simulink model "SpheroMoveToPoint"  (R2014a)
settings: Solver=ode45  StartTime=0.0  StopTime=8  RelTol=1e-3
InitFcn:
  | sphName = uint8('Sphero-PGP');
StopFcn:
  | move(sphName, 0, 0)
  | move(sphName, 0, 0, 0)
undefined symbols (not defined in the file or in its folder): Kd, Ki, Kp
libraries: simulink x5, utility x1
settings Model: Creator=dsethi  LastModifiedBy=dsethi

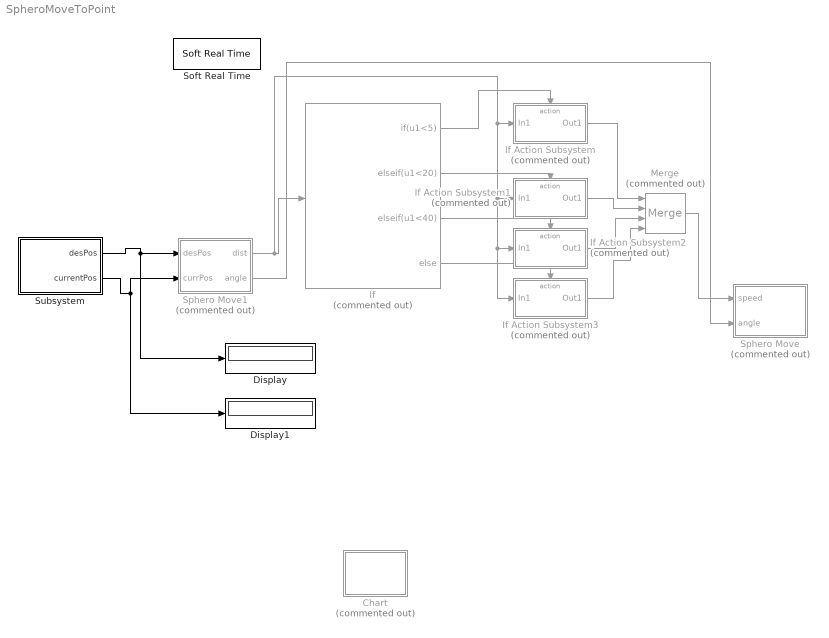
== system SpheroMoveToPoint ==
  Chart : Stateflow chart  Commented=on  TreatAsAtomicUnit=on
  Display : Display
  Display1 : Display
  If : If  Commented=on  IfExpression=u1<5  ElseIfExpressions=u1<20, u1<40
  If Action Subsystem : Subsystem  Commented=on  TreatAsAtomicUnit=on  mask{Kp=0, Ki=0, Kd=0}
  If Action Subsystem1 : Subsystem  Commented=on  TreatAsAtomicUnit=on  mask{Kp=4, Ki=0, Kd=0}
  If Action Subsystem2 : Subsystem  Commented=on  TreatAsAtomicUnit=on  mask{Kp=2, Ki=0, Kd=0}
  If Action Subsystem3 : Subsystem  Commented=on  TreatAsAtomicUnit=on  mask{Kp=0.5, Ki=0, Kd=0}
  Merge : Merge  Commented=on  Inputs=4
  Soft Real Time : utility/Soft Real Time  x=1
  Sphero Move : MATLAB Function  Commented=on  TreatAsAtomicUnit=on
  Sphero Move1 : MATLAB Function  Commented=on  TreatAsAtomicUnit=on
  Subsystem : Subsystem  mask{cameraNum=Logitech, desPos=[0, 0]}
      mask prompts: cameraNum "Camera"; desPos "Desired position (x, y coordinates)"
      mask init:
      | desPos = [0, 0]
      mask TypeOptions cameraNum: Logitech | Microsoft
  wires:
  Subsystem/1(desPos) -> Display/1, Sphero Move1/1(desPos)
  Subsystem/2(currentPos) -> Display1/1, Sphero Move1/2(currPos)
  Sphero Move1/2(angle) -> Sphero Move/2(angle)
  Sphero Move1/1(dist) -> If Action Subsystem1/1(In1), If Action Subsystem2/1(In1), If Action Subsystem3/1(In1), If Action Subsystem/1(In1), If/1
  If/1 -> If Action Subsystem/Action
  If/2 -> If Action Subsystem1/Action
  If/3 -> If Action Subsystem2/Action
  If/4 -> If Action Subsystem3/Action
  If Action Subsystem3/1(Out1) -> Merge/4
  If Action Subsystem2/1(Out1) -> Merge/3
  If Action Subsystem1/1(Out1) -> Merge/2
  If Action Subsystem/1(Out1) -> Merge/1
  Merge/1 -> Sphero Move/1(speed)

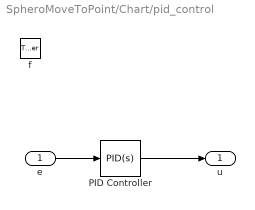
== system SpheroMoveToPoint/Chart/pid_control ==
  e : Inport  OutDataTypeStr=double  PortDimensions=1
  f : TriggerPort  TriggerType=function-call
      settings: CopyFcn=Stateflow.SLINSF.SimulinkMan.removeBlockPreDeleteFcn  PreDeleteFcn=Stateflow.SLINSF.SimulinkMan.unsafePredeleteFcn
  PID Controller : simulink/Continuous/PID Controller  Controller=PID  TimeDomain=Continuous-time  SampleTime=1  IntegratorMethod=Forward Euler  FilterMethod=Forward Euler  Form=Parallel  P=Kp  I=Ki  D=Kd  N=100  InitialConditionSource=internal  InitialConditionForIntegrator=0  InitialConditionForFilter=0  ExternalReset=none  LimitOutput=off  UpperSaturationLimit=inf  LowerSaturationLimit=-inf  LinearizeAsGain=on  AntiWindupMode=none  Kb=1  TrackingMode=off  Kt=1  PParamMin=[]  PParamMax=[]  IParamMin=[]  IParamMax=[]  DParamMin=[]  DParamMax=[]  NParamMin=[]  NParamMax=[]  KbParamMin=[]  KbParamMax=[]  KtParamMin=[]  KtParamMax=[]  POutMin=[]  POutMax=[]  IOutMin=[]  IOutMax=[]  DOutMin=[]  DOutMax=[]  NOutMin=[]  NOutMax=[]  KbOutMin=[]  KbOutMax=[]  KtOutMin=[]  KtOutMax=[]  IntegratorOutMin=[]  IntegratorOutMax=[]  FilterOutMin=[]  FilterOutMax=[]  SumOutMin=[]  SumOutMax=[]  SumI1OutMin=[]  SumI1OutMax=[]  SumI2OutMin=[]  SumI2OutMax=[]  SumI3OutMin=[]  SumI3OutMax=[]  SumDOutMin=[]  SumDOutMax=[]  SaturationOutMin=[]  SaturationOutMax=[]  IntegratorContinuousStateAttributes=''  IntegratorStateMustResolveToSignalObject=off  IntegratorRTWStateStorageClass=Auto  FilterContinuousStateAttributes=''  FilterStateMustResolveToSignalObject=off  FilterRTWStateStorageClass=Auto
  u : Outport
  wires:
  e/1 -> PID Controller/1
  PID Controller/1 -> u/1

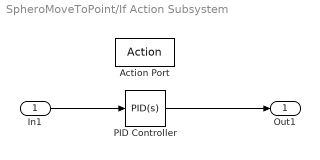
== system SpheroMoveToPoint/If Action Subsystem ==
  In1 : Inport
  Action Port : ActionPort  ActionType=then
  PID Controller : simulink/Continuous/PID Controller  Controller=PID  TimeDomain=Continuous-time  SampleTime=1  IntegratorMethod=Forward Euler  FilterMethod=Forward Euler  Form=Parallel  P=Kp  I=Ki  D=Kd  N=100  InitialConditionSource=internal  InitialConditionForIntegrator=0  InitialConditionForFilter=0  ExternalReset=none  LimitOutput=off  UpperSaturationLimit=inf  LowerSaturationLimit=-inf  LinearizeAsGain=on  AntiWindupMode=none  Kb=1  TrackingMode=off  Kt=1  PParamMin=[]  PParamMax=[]  IParamMin=[]  IParamMax=[]  DParamMin=[]  DParamMax=[]  NParamMin=[]  NParamMax=[]  KbParamMin=[]  KbParamMax=[]  KtParamMin=[]  KtParamMax=[]  POutMin=[]  POutMax=[]  IOutMin=[]  IOutMax=[]  DOutMin=[]  DOutMax=[]  NOutMin=[]  NOutMax=[]  KbOutMin=[]  KbOutMax=[]  KtOutMin=[]  KtOutMax=[]  IntegratorOutMin=[]  IntegratorOutMax=[]  FilterOutMin=[]  FilterOutMax=[]  SumOutMin=[]  SumOutMax=[]  SumI1OutMin=[]  SumI1OutMax=[]  SumI2OutMin=[]  SumI2OutMax=[]  SumI3OutMin=[]  SumI3OutMax=[]  SumDOutMin=[]  SumDOutMax=[]  SaturationOutMin=[]  SaturationOutMax=[]  IntegratorContinuousStateAttributes=''  IntegratorStateMustResolveToSignalObject=off  IntegratorRTWStateStorageClass=Auto  FilterContinuousStateAttributes=''  FilterStateMustResolveToSignalObject=off  FilterRTWStateStorageClass=Auto
  Out1 : Outport
  wires:
  PID Controller/1 -> Out1/1
  In1/1 -> PID Controller/1

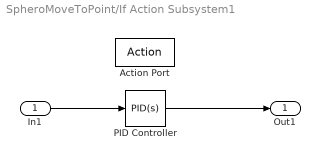
== system SpheroMoveToPoint/If Action Subsystem1 ==
  In1 : Inport
  Action Port : ActionPort  ActionType=elseif
  PID Controller : simulink/Continuous/PID Controller  Controller=PID  TimeDomain=Continuous-time  SampleTime=1  IntegratorMethod=Forward Euler  FilterMethod=Forward Euler  Form=Parallel  P=Kp  I=Ki  D=Kd  N=100  InitialConditionSource=internal  InitialConditionForIntegrator=0  InitialConditionForFilter=0  ExternalReset=none  LimitOutput=off  UpperSaturationLimit=inf  LowerSaturationLimit=-inf  LinearizeAsGain=on  AntiWindupMode=none  Kb=1  TrackingMode=off  Kt=1  PParamMin=[]  PParamMax=[]  IParamMin=[]  IParamMax=[]  DParamMin=[]  DParamMax=[]  NParamMin=[]  NParamMax=[]  KbParamMin=[]  KbParamMax=[]  KtParamMin=[]  KtParamMax=[]  POutMin=[]  POutMax=[]  IOutMin=[]  IOutMax=[]  DOutMin=[]  DOutMax=[]  NOutMin=[]  NOutMax=[]  KbOutMin=[]  KbOutMax=[]  KtOutMin=[]  KtOutMax=[]  IntegratorOutMin=[]  IntegratorOutMax=[]  FilterOutMin=[]  FilterOutMax=[]  SumOutMin=[]  SumOutMax=[]  SumI1OutMin=[]  SumI1OutMax=[]  SumI2OutMin=[]  SumI2OutMax=[]  SumI3OutMin=[]  SumI3OutMax=[]  SumDOutMin=[]  SumDOutMax=[]  SaturationOutMin=[]  SaturationOutMax=[]  IntegratorContinuousStateAttributes=''  IntegratorStateMustResolveToSignalObject=off  IntegratorRTWStateStorageClass=Auto  FilterContinuousStateAttributes=''  FilterStateMustResolveToSignalObject=off  FilterRTWStateStorageClass=Auto
  Out1 : Outport
  wires:
  In1/1 -> PID Controller/1
  PID Controller/1 -> Out1/1

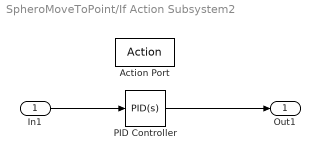
== system SpheroMoveToPoint/If Action Subsystem2 ==
  In1 : Inport
  Action Port : ActionPort  ActionType=elseif
  PID Controller : simulink/Continuous/PID Controller  Controller=PID  TimeDomain=Continuous-time  SampleTime=1  IntegratorMethod=Forward Euler  FilterMethod=Forward Euler  Form=Parallel  P=Kp  I=Ki  D=Kd  N=100  InitialConditionSource=internal  InitialConditionForIntegrator=0  InitialConditionForFilter=0  ExternalReset=none  LimitOutput=off  UpperSaturationLimit=inf  LowerSaturationLimit=-inf  LinearizeAsGain=on  AntiWindupMode=none  Kb=1  TrackingMode=off  Kt=1  PParamMin=[]  PParamMax=[]  IParamMin=[]  IParamMax=[]  DParamMin=[]  DParamMax=[]  NParamMin=[]  NParamMax=[]  KbParamMin=[]  KbParamMax=[]  KtParamMin=[]  KtParamMax=[]  POutMin=[]  POutMax=[]  IOutMin=[]  IOutMax=[]  DOutMin=[]  DOutMax=[]  NOutMin=[]  NOutMax=[]  KbOutMin=[]  KbOutMax=[]  KtOutMin=[]  KtOutMax=[]  IntegratorOutMin=[]  IntegratorOutMax=[]  FilterOutMin=[]  FilterOutMax=[]  SumOutMin=[]  SumOutMax=[]  SumI1OutMin=[]  SumI1OutMax=[]  SumI2OutMin=[]  SumI2OutMax=[]  SumI3OutMin=[]  SumI3OutMax=[]  SumDOutMin=[]  SumDOutMax=[]  SaturationOutMin=[]  SaturationOutMax=[]  IntegratorContinuousStateAttributes=''  IntegratorStateMustResolveToSignalObject=off  IntegratorRTWStateStorageClass=Auto  FilterContinuousStateAttributes=''  FilterStateMustResolveToSignalObject=off  FilterRTWStateStorageClass=Auto
  Out1 : Outport
  wires:
  PID Controller/1 -> Out1/1
  In1/1 -> PID Controller/1

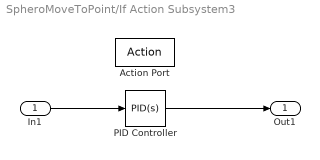
== system SpheroMoveToPoint/If Action Subsystem3 ==
  In1 : Inport
  Action Port : ActionPort  ActionType=else
  PID Controller : simulink/Continuous/PID Controller  Controller=PID  TimeDomain=Continuous-time  SampleTime=1  IntegratorMethod=Forward Euler  FilterMethod=Forward Euler  Form=Parallel  P=Kp  I=Ki  D=Kd  N=100  InitialConditionSource=internal  InitialConditionForIntegrator=0  InitialConditionForFilter=0  ExternalReset=none  LimitOutput=off  UpperSaturationLimit=inf  LowerSaturationLimit=-inf  LinearizeAsGain=on  AntiWindupMode=none  Kb=1  TrackingMode=off  Kt=1  PParamMin=[]  PParamMax=[]  IParamMin=[]  IParamMax=[]  DParamMin=[]  DParamMax=[]  NParamMin=[]  NParamMax=[]  KbParamMin=[]  KbParamMax=[]  KtParamMin=[]  KtParamMax=[]  POutMin=[]  POutMax=[]  IOutMin=[]  IOutMax=[]  DOutMin=[]  DOutMax=[]  NOutMin=[]  NOutMax=[]  KbOutMin=[]  KbOutMax=[]  KtOutMin=[]  KtOutMax=[]  IntegratorOutMin=[]  IntegratorOutMax=[]  FilterOutMin=[]  FilterOutMax=[]  SumOutMin=[]  SumOutMax=[]  SumI1OutMin=[]  SumI1OutMax=[]  SumI2OutMin=[]  SumI2OutMax=[]  SumI3OutMin=[]  SumI3OutMax=[]  SumDOutMin=[]  SumDOutMax=[]  SaturationOutMin=[]  SaturationOutMax=[]  IntegratorContinuousStateAttributes=''  IntegratorStateMustResolveToSignalObject=off  IntegratorRTWStateStorageClass=Auto  FilterContinuousStateAttributes=''  FilterStateMustResolveToSignalObject=off  FilterRTWStateStorageClass=Auto
  Out1 : Outport
  wires:
  In1/1 -> PID Controller/1
  PID Controller/1 -> Out1/1

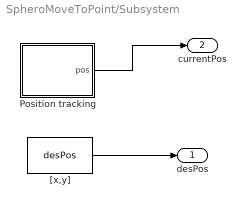
== system SpheroMoveToPoint/Subsystem ==
  Position tracking : MATLAB Function  TreatAsAtomicUnit=on
  "[x,y]" : Constant  Value=desPos
  desPos : Outport
  currentPos : Outport  Port=2
  wires:
  Position tracking/1(pos) -> currentPos/1
  "[x,y]"/1 -> desPos/1

== matlab function SpheroMoveToPoint/Subsystem/Position tracking ==
  data: pos output; cameraNum parameter
function pos = fcn(cameraNum)
%#codegen
coder.extrinsic('detectSphero')
pos = [0, 0];

if isempty(cameraNum)||~(cameraNum==1||cameraNum==2)
    pos = detectSphero();
else
    pos = detectSphero(cameraNum);
end

== matlab function SpheroMoveToPoint/Sphero Move ==
  data: speed input; angle input; sphName parameter uint8
function fcn(speed, angle, sphName)
%#codegen
coder.extrinsic('move')

move(char(sphName), speed, angle);

== matlab function SpheroMoveToPoint/Sphero Move1 ==
  data: desPos input; currPos input uint8; dist output; angle output
function [dist, angle] = fcn(desPos, currPos)
%#codegen
if currPos(1)<0 || currPos(2)<0
    dist = Inf;
    return
end
%% Angle and distance calculation
 
    %Angle of desired position wrt y axis (or orientation of sphero)
    angle = atan2(desPos(1)-currPos(1), desPos(2)-currPos(2));

    if angle<0
        angle = -angle;
    else
        angle = 2*pi-angle;
    end

    angle = rad2deg(angle);

    dist = pdist([desPos; currPos]); %Distance or the error

== stateflow chart SpheroMoveToPoint/Chart ==
  state CloseControl
  state u = pid_control(e) [function]
  state CloseControl1
  (default) -> CloseControl
  data: desPos function_input; currPos function_input; dist function_output; angle function_output; e function_input double size=1; u function_output
  function [dist, angle] = relativePos(desPos, currPos):
    | function [dist, angle] = relativePos(desPos, currPos)
    | if currPos(1)<0 || currPos(2)<0
    |     dist = Inf;
    |     return
    | end
    | %% Angle and distance calculation
    |  
    |     %Angle of desired position wrt y axis (or orientation of sphero)
    |     angle = atan2(desPos(1)-currPos(1), desPos(2)-currPos(2));
    | 
    |     if angle<0
    |         angle = -angle;
    |     else
    |         angle = 2*pi-angle;
    |     end
    | 
    |     angle = rad2deg(angle);
    | 
    |     dist = pdist([desPos; currPos]); %Distance or the error
